simulink model "GPCA_INFUSION_MGR"  (Simulink 8.7)
settings: Solver=VariableStepAuto  StartTime=0.0  StopTime=10.0  RelTol=1e-3
model workspace (MAT data in the model file):
  input_struct.time = [0; 1; 2; 3; 4; 5; 6; 7; 8; 9; 10; 11; 12; 13; 14; 15; 16; 17; 18; 19; 20; 21; 22; 23; 24; 25; 26; 27; 28; 29; 30; 31; 32; 33; 34; 35; 36; 37; 38; 39; 40; 41; 42; 43; 44; 45; 46; 47; 48; 49; 50; 51; 52; 53; 54; 55; 56; 57; 58; 59; 60; 61; 62; 63; 64; 65; 66; 67; 68; 69; 70; 71; 72; 73; 74; 75; 76; 77; 78; 79; 80; 81; 82; 83; 84; 85; 86; 87; 88; 89; 90; 91; 92; 93; 94; 95; 96; 97; 98; 99; 100]
  input_struct.signals(1).name = 'Sys_On'
  input_struct.signals(1).values = [1; 1; 1; 1; 1; 1; 1; 1; 1; 1; 1; 1; 1; 1; 1; 1; 1; 1; 1; 1; 1; 1; 1; 1; 1; 1; 1; 1; 1; 1; 1; 1; 1; 1; 1; 1; 1; 1; 1; 1; 1; 1; 1; 1; 1; 1; 1; 1; 1; 1; 1; 1; 1; 1; 1; 1; 1; 1; 1; 1; 1; 1; 1; 1; 1; 1; 1; 1; 1; 1; 1; 1; 1; 1; 1; 1; 1; 1; 1; 1; 1; 1; 1; 1; 1; 1; 1; 1; 1; 1; 1; 1; 1; 1; 1; 1; 1; 1; 1; 1; 1]
  input_struct.signals(1).dimensions = 1
  input_struct.signals(2).name = 'Infusion_initial'
  input_struct.signals(2).values = [1; 1; 1; 1; 1; 1; 1; 1; 1; 1; 1; 1; 1; 1; 1; 1; 1; 1; 1; 1; 1; 1; 1; 1; 1; 1; 1; 1; 1; 1; 1; 1; 1; 1; 1; 1; 1; 1; 1; 1; 1; 1; 1; 1; 1; 1; 1; 1; 1; 1; 1; 1; 1; 1; 1; 1; 1; 1; 1; 1; 1; 1; 1; 1; 1; 1; 1; 1; 1; 1; 1; 1; 1; 1; 1; 1; 1; 1; 1; 1; 1; 1; 1; 1; 1; 1; 1; 1; 1; 1; 1; 1; 1; 1; 1; 1; 1; 1; 1; 1; 1]
  input_struct.signals(2).dimensions = 1
  input_struct.signals(3).name = 'In3'
  input_struct.signals(3).values = [1; 1; 1; 1; 1; 1; 1; 1; 1; 1; 1; 1; 1; 1; 1; 1; 1; 1; 1; 1; 1; 1; 1; 1; 1; 1; 1; 1; 1; 1; 1; 1; 1; 1; 1; 1; 1; 1; 1; 1; 1; 1; 1; 1; 1; 1; 1; 1; 1; 1; 1; 1; 1; 1; 1; 1; 1; 1; 1; 1; 1; 1; 1; 1; 1; 1; 1; 1; 1; 1; 1; 1; 1; 1; 1; 1; 1; 1; 1; 1; 1; 1; 1; 1; 1; 1; 1; 1; 1; 1; 1; 1; 1; 1; 1; 1; 1; 1; 1; 1; 1]
  input_struct.signals(3).dimensions = 1
  input_struct.signals(4).name = 'In4'
  input_struct.signals(4).values = [1; 1; 1; 1; 1; 1; 1; 1; 1; 1; 1; 1; 1; 1; 1; 1; 1; 1; 1; 1; 1; 1; 1; 1; 1; 1; 1; 1; 1; 1; 1; 1; 1; 1; 1; 1; 1; 1; 1; 1; 1; 1; 1; 1; 1; 1; 1; 1; 1; 1; 1; 1; 1; 1; 1; 1; 1; 1; 1; 1; 1; 1; 1; 1; 1; 1; 1; 1; 1; 1; 1; 1; 1; 1; 1; 1; 1; 1; 1; 1; 1; 1; 1; 1; 1; 1; 1; 1; 1; 1; 1; 1; 1; 1; 1; 1; 1; 1; 1; 1; 1]
  input_struct.signals(4).dimensions = 1
  input_struct.signals(5).name = 'In5'
  input_struct.signals(5).values = [1; 1; 1; 1; 1; 1; 1; 1; 1; 1; 1; 1; 1; 1; 1; 1; 1; 1; 1; 1; 1; 1; 1; 1; 1; 1; 1; 1; 1; 1; 1; 1; 1; 1; 1; 1; 1; 1; 1; 1; 1; 1; 1; 1; 1; 1; 1; 1; 1; 1; 1; 1; 1; 1; 1; 1; 1; 1; 1; 1; 1; 1; 1; 1; 1; 1; 1; 1; 1; 1; 1; 1; 1; 1; 1; 1; 1; 1; 1; 1; 1; 1; 1; 1; 1; 1; 1; 1; 1; 1; 1; 1; 1; 1; 1; 1; 1; 1; 1; 1; 1]
  input_struct.signals(5).dimensions = 1
  input_struct.signals(6).name = 'In6'
  input_struct.signals(6).values = [44; 62; 24; 71; 99; 17; 64; 65; 64; 99; 39; 27; 46; 12; 36; 79; 31; 74; 65; 84; 53; 39; 62; 61; 54; 74; 38; 13; 37; 82; 90; 35; 2; 3; 85; 94; 77; 97; 50; 56; 66; 98; 91; 3; 58; 73; 16; 5; 54; 4; 50; 22; 48; 66; 5; 86; 4; 65; 51; 58; 88; 19; 21; 14; 83; 74; 90; 16; 43; 63; 60; 30; 79; 39; 99; 21; 78; 85; 47; 68; 80; 24; 76; 93; 100; 89; 51; 1; 2; 10; 79; 56; 72; 23; 2; 13; 64; 2; 95; 100; 38]
  input_struct.signals(6).dimensions = 1
  input_struct.signals(7).name = 'In7'
  input_struct.signals(7).values = [90; 60; 84; 49; 6; 47; 32; 92; 90; 66; 25; 24; 55; 40; 76; 40; 27; 35; 94; 38; 49; 24; 54; 22; 30; 54; 51; 50; 92; 74; 90; 81; 45; 24; 7; 29; 44; 46; 98; 93; 60; 59; 12; 40; 95; 22; 18; 35; 63; 44; 42; 29; 91; 69; 11; 9; 2; 92; 37; 43; 58; 19; 3; 66; 46; 20; 20; 70; 75; 55; 53; 41; 56; 74; 30; 79; 8; 48; 40; 92; 43; 95; 41; 25; 88; 50; 43; 56; 25; 26; 21; 59; 84; 86; 65; 99; 98; 69; 79; 35; 79]
  input_struct.signals(7).dimensions = 1
  input_struct.signals(8).name = 'In8'
  input_struct.signals(8).values = [4.63973383023; 35.2832639735; 35.6997824976; 12.9735038436; 98.2246278024; 41.5753843769; 40.648526584; 78.2690731191; 43.3204076201; 57.6278133584; 65.0468332085; 3.301078952; 40.4011686703; 95.8944237105; 59.5519789208; 93.3078447207; 93.7040801805; 75.5739132103; 53.8914185396; 82.4291331591; 1.07468467942; 74.6518961279; 10.3034771476; 4.84107839062; 18.5691118817; 47.2839709594; 0.963562412951; 85.8180487504; 47.3489526284; 14.9934750248; 24.5454645634; 5.6791143473; 20.524479776; 46.5489139189; 46.0975178173; 35.1056074586; 44.1002771924; 32.9407034078; 57.2097266663; 99.2353294257; 71.7850824726; 36.0995549494; 57.2728531087; 38.0334616232; 37.2083265954; 42.4274644079; 74.3126890424; 36.008048598; 62.64892526; 85.2869697994; 12.0024751155; 17.4342661023; 95.0627797395; 97.7501474465; 25.200487502; 28.4620466338; 83.8286322237; 80.2100740647; 36.9961325274; 36.2810980898; 27.1741280369; 25.946930682; 99.4394376478; 4.6263321519; 67.6333122761; 50.1684647694; 11.3288004525; 46.1314661009; 71.8630508731; 96.0602806974; 52.8900107169; 93.5416699007; 98.9586946718; 46.5715874257; 36.3796463512; 9.03358580397; 84.4203757713; 41.3706063981; 75.7358446323; 55.4033391719; 47.6240269519; 26.6590463476; 13.5277473048; 7.77007824224; 84.6593448102; 33.7042967675; 67.3993808562; 10.4432752721; 58.7365871172; 11.4802921597; 24.9345347125; 41.4172719483; 71.5466741055; 86.9670580513; 81.5427904751; 23.2449226705; 34.6335232103; 96.0612364005; 30.1312799866; 15.4196271404; 74.4436488973]
  input_struct.signals(8).dimensions = 1
  input_struct.signals(9).name = 'In9'
  input_struct.signals(9).values = [29; 33; 1; 57; 45; 17; 71; 55; 26; 40; 25; 59; 6; 61; 4; 87; 35; 12; 60; 64; 79; 74; 80; 65; 92; 61; 74; 72; 69; 92; 97; 33; 10; 81; 69; 18; 49; 94; 14; 66; 20; 63; 63; 45; 66; 45; 86; 71; 43; 63; 65; 89; 100; 73; 51; 5; 11; 86; 92; 68; 47; 97; 8; 39; 2; 60; 57; 2; 59; 37; 3; 98; 14; 56; 87; 69; 4; 45; 44; 77; 100; 26; 89; 5; 34; 73; 50; 55; 23; 13; 49; 88; 65; 45; 14; 15; 99; 98; 43; 76; 56]
  input_struct.signals(9).dimensions = 1
  input_struct.signals(10).name = 'In10'
  input_struct.signals(10).values = [75.6654394055; 97.5920093113; 4.18740489107; 35.1003499457; 47.6647962675; 17.4935331391; 35.5904543428; 88.8469466736; 6.915304919; 9.27474343383; 20.580418117; 61.5198979774; 27.3432050518; 74.7785372302; 30.5726330316; 76.5444360829; 25.2885731381; 67.1015975406; 13.1914107685; 94.2448397517; 44.4583183004; 35.7995338956; 16.9800958046; 49.9074065297; 45.2166200379; 6.62159801851; 88.788167464; 90.7784125901; 78.2654328509; 47.1943559213; 79.6142303751; 87.5647388455; 67.2251562171; 7.03827356925; 12.4471905164; 42.5366183349; 78.2665768727; 58.9146545218; 47.2135906387; 3.37884713121; 18.0073535626; 93.1819658789; 59.0764009202; 50.63355074; 21.8438856709; 95.205103594; 36.2259513867; 45.8546754703; 83.0810137982; 79.0665029294; 44.1022733276; 62.4033793782; 95.5508256318; 66.3478658469; 26.6490943364; 72.3154840215; 56.1077886344; 97.2980667354; 30.0872644671; 49.7020498287; 28.3954108418; 7.42080047907; 11.1397187358; 7.53069359706; 99.6192027606; 59.9597679943; 78.8968013382; 86.1268639612; 82.7068266283; 93.6923731938; 3.58534605987; 13.9710786829; 72.5442080874; 87.2094169044; 37.4103271527; 21.6187517238; 57.6010099173; 2.56467550787; 4.35049245994; 93.3449284046; 40.1651928267; 78.4920768198; 24.2628568325; 60.8542724961; 89.3183909504; 62.9419861275; 92.4146871352; 99.5804571701; 15.0089872708; 2.47968997642; 91.1264097869; 14.7997458476; 8.99430572891; 71.5693599151; 17.5014408721; 15.9721590177; 47.8932143834; 94.8731651593; 74.1070141458; 67.2333462131; 7.03452477692]
  input_struct.signals(10).dimensions = 1
  input_struct.signals(11).name = 'In11'
  input_struct.signals(11).values = [30.6105485336; 93.6833055516; 85.6937003671; 89.0847380737; 58.8586918838; 16.2586327547; 17.6045119807; 74.7563614666; 94.5285815976; 65.7979789003; 54.3831976949; 59.7653088285; 23.4602892008; 81.9767731385; 78.8495533289; 58.9059613176; 43.6259778173; 54.973942777; 35.2968705936; 99.5791193529; 36.4963600016; 96.6174491518; 2.47408729527; 77.7839114133; 44.0182119351; 63.0499928301; 31.4024696203; 92.1815284508; 22.3324620519; 37.4486271858; 30.8144382373; 3.78224741229; 60.5169674512; 83.586436936; 58.8252232814; 36.3454795409; 13.988518362; 11.6533721537; 98.1217434069; 54.169234903; 8.65099084385; 25.6096227789; 20.9775010836; 31.4609803605; 90.3751596102; 52.0696307127; 16.2236010012; 14.3612207513; 6.40530754781; 85.4645458624; 97.4456785593; 92.9025103555; 40.9520221274; 90.1611220035; 48.4497228782; 46.9673840237; 16.7828198886; 8.28584731024; 63.3161255034; 31.0978917444; 46.6354034749; 21.1069421813; 0.14457196441; 79.7611265023; 36.8047426089; 1.513757221; 71.497846647; 21.8578762078; 68.8717269625; 24.6007221266; 26.6084854589; 13.2070823774; 34.4210335433; 75.4389983788; 88.9238646635; 71.0436376648; 24.647502524; 45.1389348495; 93.1224274285; 61.5667580202; 25.8289980493; 63.1103174057; 69.5532194169; 40.3659878092; 19.3481857413; 30.7074224713; 69.2954513388; 63.0359565476; 24.9823988841; 4.34220177336; 53.1451453615; 17.6201447979; 52.1902037473; 87.1282135693; 61.3612826085; 27.1432121467; 85.453961022; 15.7460139606; 25.941863813; 67.0580480613; 22.5957392867]
  input_struct.signals(11).dimensions = 1
  input_struct.signals(12).name = 'In12'
  input_struct.signals(12).values = [83; 33; 49; 77; 74; 64; 25; 74; 34; 31; 13; 2; 93; 92; 39; 71; 68; 13; 21; 91; 90; 38; 26; 61; 63; 2; 82; 52; 91; 12; 95; 93; 10; 42; 33; 85; 95; 73; 69; 65; 32; 74; 16; 77; 10; 97; 61; 90; 20; 99; 25; 23; 41; 79; 84; 41; 41; 78; 25; 87; 69; 98; 19; 22; 32; 76; 37; 61; 39; 56; 39; 67; 2; 82; 35; 72; 96; 51; 67; 43; 85; 66; 51; 37; 69; 10; 5; 87; 66; 62; 43; 51; 17; 10; 69; 15; 53; 1; 43; 23; 66]
  input_struct.signals(12).dimensions = 1
  input_struct.signals(13).name = 'In13'
  input_struct.signals(13).values = [50.310189638; 60.0057239808; 20.017365886; 13.7401018724; 2.37890286344; 93.9542698221; 69.550132379; 55.4233183009; 29.5414289119; 4.26317475057; 85.3760208334; 59.6682100841; 1.85267796429; 93.3190961871; 0.978832426687; 64.0955539628; 78.8685383549; 52.6502944231; 29.1248417281; 62.8328540884; 42.5468671552; 54.6370363273; 19.0797083319; 74.448883701; 21.2856219278; 10.0122455877; 89.6384986298; 82.2336975388; 88.278375005; 8.81242954122; 70.0187647741; 17.022422373; 83.3044271053; 72.8057084722; 77.5893015136; 76.3495251449; 5.70994655747; 60.9847721619; 89.8471800448; 51.6130724509; 50.6171538067; 25.5616556411; 97.1603134959; 58.1123922451; 96.8386414337; 4.14383729209; 18.8628229362; 51.9760059068; 64.0853919663; 34.0731322525; 64.8329819208; 35.5437965546; 85.0430024041; 54.2804681241; 67.3080087461; 25.6572579313; 12.1338276708; 4.06064458603; 88.7943133089; 75.3187315832; 80.2079185026; 44.1405626647; 7.51725857162; 15.4229697288; 24.7244148394; 7.92259868541; 85.3159563134; 15.7176855291; 61.6662683689; 52.8449944459; 19.1219823356; 75.9750760227; 61.4998425493; 15.2063606777; 45.4637446858; 68.2097599809; 28.1259121576; 62.4863120815; 94.1730122601; 56.6803336047; 69.3115599105; 97.8586411034; 89.9117378675; 64.8479896015; 98.2920814945; 16.381496818; 50.9786857228; 62.7348429656; 80.0000906333; 41.7769086107; 5.48344318938; 51.9144193651; 13.4532135688; 36.6974434645; 69.6620887403; 12.9583524717; 78.5849529987; 5.03089735964; 81.5615519701; 86.6938862459; 19.6896453654]
  input_struct.signals(13).dimensions = 1
  input_struct.signals(14).name = 'In14'
  input_struct.signals(14).values = [60.7393801127; 99.6679751886; 4.23743274601; 13.8823003129; 22.2953974091; 58.3010477964; 67.1106486856; 72.3195985118; 50.4438512986; 64.4630262831; 3.6369340676; 19.3851825335; 74.9545712103; 30.8178375845; 74.9052151825; 85.2037321352; 9.93554763828; 59.7778198788; 72.0602255764; 56.8713832115; 23.5110091085; 91.0636226409; 95.0619757095; 51.631529482; 70.7088130257; 79.879519294; 19.9689366653; 10.684051545; 61.8574843316; 2.22239407823; 3.75620436883; 11.5364121588; 81.8697240446; 37.6899225803; 22.9156312136; 36.8139913037; 17.4540423871; 77.4779638833; 33.0030614354; 31.5780139928; 72.4586900626; 58.4954983442; 77.7755524267; 35.9576387651; 18.4733001916; 57.3689108129; 48.3094584565; 42.1626940454; 31.7325192381; 97.2571507193; 25.8222640837; 56.7099899646; 35.2066904741; 31.202960892; 0.939760275739; 66.8127492036; 88.5687680497; 42.1317726472; 85.8580052735; 94.7992491693; 37.6106774797; 20.329324849; 17.9169495241; 30.6294083341; 85.0311935666; 52.5602531045; 82.844225188; 10.6876458874; 61.71420317; 56.6826518566; 26.0936156907; 0.230811043294; 28.725506288; 82.1270082457; 89.511540468; 99.5807909606; 0.843840180703; 73.284323844; 8.46172679425; 63.3348568099; 80.5086425609; 82.9964886435; 56.7221449724; 26.0043390493; 78.4532049402; 16.9205334021; 27.4258345175; 0.490319428856; 39.7561240528; 2.65515532308; 85.469904981; 20.4891689163; 86.0350581098; 5.61247088055; 22.3511772366; 4.52805178084; 75.0991773113; 69.805637993; 91.8787889121; 90.8922604332; 80.5523856545]
  input_struct.signals(14).dimensions = 1
  input_struct.signals(15).name = 'In15'
  input_struct.signals(15).values = [100; 81; 33; 3; 74; 48; 40; 87; 6; 39; 15; 5; 70; 92; 39; 25; 91; 71; 90; 95; 94; 100; 40; 66; 83; 63; 71; 49; 51; 78; 5; 91; 74; 62; 76; 29; 21; 66; 93; 81; 36; 28; 75; 73; 86; 92; 27; 69; 62; 8; 19; 34; 32; 43; 9; 56; 67; 12; 32; 99; 89; 3; 87; 25; 44; 14; 22; 78; 9; 41; 60; 20; 70; 60; 47; 25; 42; 78; 4; 61; 8; 42; 99; 85; 6; 73; 12; 49; 87; 2; 82; 79; 20; 92; 69; 89; 72; 49; 84; 10; 3]
  input_struct.signals(15).dimensions = 1
  input_struct.signals(16).name = 'In16'
  input_struct.signals(16).values = [34; 49; 23; 56; 69; 84; 90; 44; 40; 45; 31; 45; 97; 47; 50; 3; 20; 90; 39; 11; 35; 18; 25; 65; 98; 93; 6; 91; 19; 100; 33; 23; 95; 82; 93; 72; 88; 87; 36; 14; 81; 69; 44; 95; 96; 4; 28; 7; 83; 40; 59; 35; 98; 61; 67; 87; 43; 8; 88; 70; 85; 68; 71; 90; 59; 33; 100; 21; 29; 84; 78; 21; 77; 62; 97; 51; 48; 59; 98; 35; 27; 59; 75; 9; 38; 9; 32; 46; 17; 6; 45; 29; 20; 51; 2; 84; 21; 43; 74; 53; 27]
  input_struct.signals(16).dimensions = 1
  input_struct.signals(17).name = 'In17'
  input_struct.signals(17).values = [77; 96; 12; 3; 43; 7; 13; 10; 24; 22; 61; 40; 73; 97; 76; 8; 87; 37; 80; 79; 34; 95; 83; 63; 30; 62; 99; 35; 24; 1; 91; 63; 79; 75; 62; 19; 85; 72; 66; 62; 88; 80; 73; 41; 100; 63; 36; 19; 33; 26; 95; 90; 99; 96; 88; 17; 15; 65; 80; 8; 25; 2; 24; 26; 92; 37; 4; 66; 82; 9; 2; 37; 42; 42; 47; 47; 55; 54; 51; 79; 29; 56; 58; 21; 56; 22; 55; 7; 87; 21; 24; 39; 29; 76; 32; 11; 81; 26; 51; 4; 63]
  input_struct.signals(17).dimensions = 1
  input_struct.signals(18).name = 'In18'
  input_struct.signals(18).values = [39; 31; 34; 94; 47; 1; 73; 40; 3; 64; 44; 60; 62; 46; 5; 72; 75; 41; 6; 95; 88; 83; 45; 89; 86; 65; 51; 8; 37; 24; 87; 64; 74; 16; 95; 41; 62; 80; 69; 1; 51; 99; 1; 5; 11; 61; 5; 43; 36; 70; 37; 33; 68; 59; 25; 38; 21; 26; 85; 43; 66; 54; 94; 34; 37; 75; 87; 3; 85; 81; 55; 44; 61; 34; 78; 10; 46; 77; 63; 1; 2; 46; 23; 38; 45; 7; 37; 38; 31; 92; 48; 19; 30; 83; 62; 67; 62; 27; 88; 1; 37]
  input_struct.signals(18).dimensions = 1
  input_struct.signals(19).name = 'In19'
  input_struct.signals(19).values = [1; 1; 1; 1; 1; 1; 1; 1; 1; 1; 1; 1; 1; 1; 1; 1; 1; 1; 1; 1; 1; 1; 1; 1; 1; 1; 1; 1; 1; 1; 1; 1; 1; 1; 1; 1; 1; 1; 1; 1; 1; 1; 1; 1; 1; 1; 1; 1; 1; 1; 1; 1; 1; 1; 1; 1; 1; 1; 1; 1; 1; 1; 1; 1; 1; 1; 1; 1; 1; 1; 1; 1; 1; 1; 1; 1; 1; 1; 1; 1; 1; 1; 1; 1; 1; 1; 1; 1; 1; 1; 1; 1; 1; 1; 1; 1; 1; 1; 1; 1; 1]
  input_struct.signals(19).dimensions = 1
  input_struct.signals(20).name = 'In20'
  input_struct.signals(20).values = [45; 15; 66; 68; 75; 31; 81; 30; 28; 28; 77; 32; 36; 68; 4; 16; 43; 22; 77; 65; 84; 21; 44; 74; 11; 45; 50; 70; 94; 16; 6; 61; 25; 56; 68; 47; 66; 81; 86; 72; 27; 30; 19; 60; 78; 10; 41; 64; 77; 52; 5; 45; 79; 100; 85; 6; 77; 73; 76; 21; 33; 60; 98; 46; 50; 98; 77; 98; 21; 4; 16; 72; 78; 65; 34; 66; 5; 87; 11; 95; 38; 14; 32; 90; 79; 20; 18; 90; 78; 80; 22; 20; 65; 12; 51; 69; 16; 38; 81; 91; 17]
  input_struct.signals(20).dimensions : numeric (value not decoded)
libraries: simulink x12
settings Model: Creator=bourbouh  LastModifiedBy=bourbouh
settings DataIOCC: LimitDataPoints=off  SaveFormat=Dataset
settings DebuggingCC: UnderspecifiedInitializationDetection=Simplified  MergeDetectMultiDrivingBlocksExec=error
settings HardwareCC: ProdBitPerPointer=64  ProdLargestAtomicFloat=Float  ProdIntDivRoundTo=Zero  ProdEndianess=LittleEndian  ProdWordSize=64  ProdHWDeviceType=Intel->x86-64 (Windows64)
settings ModelReferenceCC: PropagateSignalLabelsOutOfModel=on
settings ConfigComp: CovModelRefEnable=off

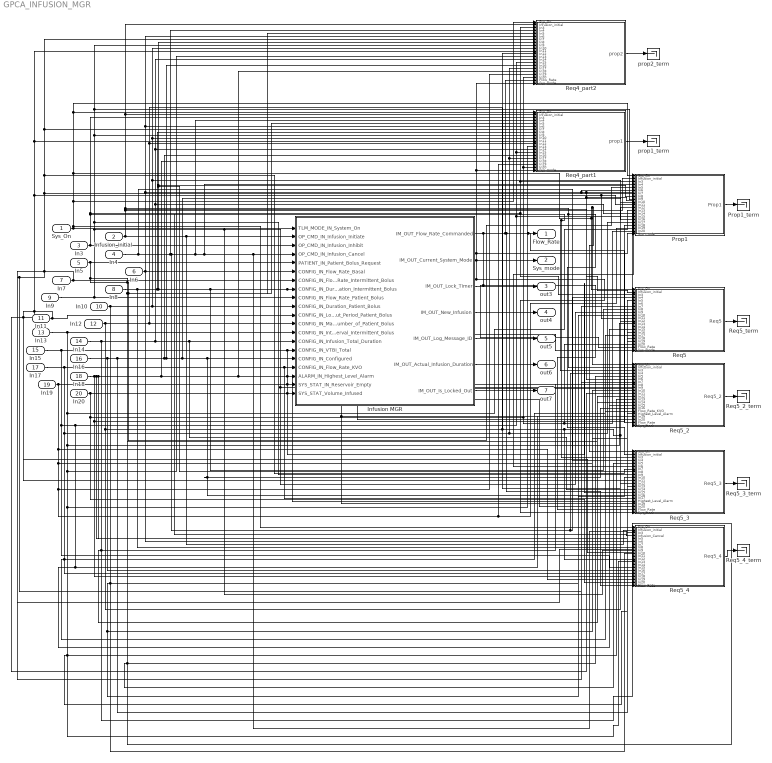
== system GPCA_INFUSION_MGR ==
  Sys_On : Inport
  Infusion_initial : Inport  Port=2
  In3 : Inport  Port=3
  In4 : Inport  Port=4
  In5 : Inport  Port=5
  In6 : Inport  Port=6
  In7 : Inport  Port=7
  In8 : Inport  Port=8
  In9 : Inport  Port=9
  In10 : Inport  Port=10
  In11 : Inport  Port=11
  In12 : Inport  Port=12
  In13 : Inport  Port=13
  In14 : Inport  Port=14
  In15 : Inport  Port=15
  In16 : Inport  Port=16
  In17 : Inport  Port=17
  In18 : Inport  Port=18
  In19 : Inport  Port=19
  In20 : Inport  Port=20
  Infusion MGR : Stateflow chart  TreatAsAtomicUnit=on
  Prop1 : Subsystem  TreatAsAtomicUnit=on  mask(Observer){AnnotationType=ensures, ObserverType=[]}
      mask prompts: AnnotationType "Type of annotation (pre/post...)"; ObserverType "Observer type"
      mask help:
      | Set an observer for the system.
      | The annotation type parameter sets the type of observer:
      | - requires : pre-condition
      | - ensures : post-condition
      | - assert : an assertion
      | - observer : the observer computes a special type of properties
      mask TypeOptions AnnotationType: ensures | requires | assert | observer
      mask Callback AnnotationType:
      | paramStr = get_param(gcb, 'MaskValues');
      | if strcmp(paramStr{1}(1),'o')
      | set_param(gcb,'MaskVisibilities',{'on';'on'});
      | paramStr{2} = 'ellipsoid';
      | set_param(gcb,'MaskValues',paramStr);
      | else
      | set_param(gcb,'MaskVisibilities',{'on';'off'});
      | end
      | clear paramStr;
      mask Callback ObserverType:
      | paramStr = get_param(gcb, 'MaskValues');
      | if strcmp(paramStr{1}(1),'o')
      | set_param(gcb,'MaskVisibilities',{'on';'on'});
      | paramStr{2} = 'ellipsoid';
      | set_param(gcb,'MaskValues',paramStr);
      | else
      | set_param(gcb,'MaskVisibilities',{'on';'off'});
      | end
      | clear paramStr;
      mask Display:
      | color('black')
      | text(0.5, 0.5, ['Property: ''' get_param(gcb,'name') ''''], 'horizontalAlignment', 'center');
      | text(0.99, 0.03, '{\bf\fontsize{12}SAFE}', 'hor', 'right', 'ver', 'bottom', 'texmode', 'on');
  Prop1_term : Terminator
  Req4_part1 : Subsystem  TreatAsAtomicUnit=on  mask(Observer){AnnotationType=ensures, ObserverType=[]}
      mask prompts: AnnotationType "Type of annotation (pre/post...)"; ObserverType "Observer type"
      mask help:
      | Set an observer for the system.
      | The annotation type parameter sets the type of observer:
      | - requires : pre-condition
      | - ensures : post-condition
      | - assert : an assertion
      | - observer : the observer computes a special type of properties
      mask TypeOptions AnnotationType: ensures | requires | assert | observer
      mask Callback AnnotationType:
      | paramStr = get_param(gcb, 'MaskValues');
      | if strcmp(paramStr{1}(1),'o')
      | set_param(gcb,'MaskVisibilities',{'on';'on'});
      | paramStr{2} = 'ellipsoid';
      | set_param(gcb,'MaskValues',paramStr);
      | else
      | set_param(gcb,'MaskVisibilities',{'on';'off'});
      | end
      | clear paramStr;
      mask Callback ObserverType:
      | paramStr = get_param(gcb, 'MaskValues');
      | if strcmp(paramStr{1}(1),'o')
      | set_param(gcb,'MaskVisibilities',{'on';'on'});
      | paramStr{2} = 'ellipsoid';
      | set_param(gcb,'MaskValues',paramStr);
      | else
      | set_param(gcb,'MaskVisibilities',{'on';'off'});
      | end
      | clear paramStr;
      mask Display:
      | color('black')
      | text(0.5, 0.5, ['Property: ''' get_param(gcb,'name') ''''], 'horizontalAlignment', 'center');
      | text(0.99, 0.03, '{\bf\fontsize{12}SAFE}', 'hor', 'right', 'ver', 'bottom', 'texmode', 'on');
  Req4_part2 : Subsystem  TreatAsAtomicUnit=on  mask(Observer){AnnotationType=ensures, ObserverType=[]}
      mask prompts: AnnotationType "Type of annotation (pre/post...)"; ObserverType "Observer type"
      mask help:
      | Set an observer for the system.
      | The annotation type parameter sets the type of observer:
      | - requires : pre-condition
      | - ensures : post-condition
      | - assert : an assertion
      | - observer : the observer computes a special type of properties
      mask TypeOptions AnnotationType: ensures | requires | assert | observer
      mask Callback AnnotationType:
      | paramStr = get_param(gcb, 'MaskValues');
      | if strcmp(paramStr{1}(1),'o')
      | set_param(gcb,'MaskVisibilities',{'on';'on'});
      | paramStr{2} = 'ellipsoid';
      | set_param(gcb,'MaskValues',paramStr);
      | else
      | set_param(gcb,'MaskVisibilities',{'on';'off'});
      | end
      | clear paramStr;
      mask Callback ObserverType:
      | paramStr = get_param(gcb, 'MaskValues');
      | if strcmp(paramStr{1}(1),'o')
      | set_param(gcb,'MaskVisibilities',{'on';'on'});
      | paramStr{2} = 'ellipsoid';
      | set_param(gcb,'MaskValues',paramStr);
      | else
      | set_param(gcb,'MaskVisibilities',{'on';'off'});
      | end
      | clear paramStr;
      mask Display:
      | color('black')
      | text(0.5, 0.5, ['Property: ''' get_param(gcb,'name') ''''], 'horizontalAlignment', 'center');
      | text(0.99, 0.03, '{\bf\fontsize{12}TIMEOUT}', 'hor', 'right', 'ver', 'bottom', 'texmode', 'on');
  Req5 : Subsystem  TreatAsAtomicUnit=on  mask(Observer){AnnotationType=ensures, ObserverType=[]}
      mask prompts: AnnotationType "Type of annotation (pre/post...)"; ObserverType "Observer type"
      mask help:
      | Set an observer for the system.
      | The annotation type parameter sets the type of observer:
      | - requires : pre-condition
      | - ensures : post-condition
      | - assert : an assertion
      | - observer : the observer computes a special type of properties
      mask TypeOptions AnnotationType: ensures | requires | assert | observer
      mask Callback AnnotationType:
      | paramStr = get_param(gcb, 'MaskValues');
      | if strcmp(paramStr{1}(1),'o')
      | set_param(gcb,'MaskVisibilities',{'on';'on'});
      | paramStr{2} = 'ellipsoid';
      | set_param(gcb,'MaskValues',paramStr);
      | else
      | set_param(gcb,'MaskVisibilities',{'on';'off'});
      | end
      | clear paramStr;
      mask Callback ObserverType:
      | paramStr = get_param(gcb, 'MaskValues');
      | if strcmp(paramStr{1}(1),'o')
      | set_param(gcb,'MaskVisibilities',{'on';'on'});
      | paramStr{2} = 'ellipsoid';
      | set_param(gcb,'MaskValues',paramStr);
      | else
      | set_param(gcb,'MaskVisibilities',{'on';'off'});
      | end
      | clear paramStr;
      mask Display:
      | color('black')
      | text(0.5, 0.5, ['Property: ''' get_param(gcb,'name') ''''], 'horizontalAlignment', 'center');
      | text(0.99, 0.03, '{\bf\fontsize{12}SAFE}', 'hor', 'right', 'ver', 'bottom', 'texmode', 'on');
  Req5_2 : Subsystem  TreatAsAtomicUnit=on  mask(Observer){AnnotationType=ensures, ObserverType=[]}
      mask prompts: AnnotationType "Type of annotation (pre/post...)"; ObserverType "Observer type"
      mask help:
      | Set an observer for the system.
      | The annotation type parameter sets the type of observer:
      | - requires : pre-condition
      | - ensures : post-condition
      | - assert : an assertion
      | - observer : the observer computes a special type of properties
      mask TypeOptions AnnotationType: ensures | requires | assert | observer
      mask Callback AnnotationType:
      | paramStr = get_param(gcb, 'MaskValues');
      | if strcmp(paramStr{1}(1),'o')
      | set_param(gcb,'MaskVisibilities',{'on';'on'});
      | paramStr{2} = 'ellipsoid';
      | set_param(gcb,'MaskValues',paramStr);
      | else
      | set_param(gcb,'MaskVisibilities',{'on';'off'});
      | end
      | clear paramStr;
      mask Callback ObserverType:
      | paramStr = get_param(gcb, 'MaskValues');
      | if strcmp(paramStr{1}(1),'o')
      | set_param(gcb,'MaskVisibilities',{'on';'on'});
      | paramStr{2} = 'ellipsoid';
      | set_param(gcb,'MaskValues',paramStr);
      | else
      | set_param(gcb,'MaskVisibilities',{'on';'off'});
      | end
      | clear paramStr;
      mask Display:
      | color('black')
      | text(0.5, 0.5, ['Property: ''' get_param(gcb,'name') ''''], 'horizontalAlignment', 'center');
      | text(0.99, 0.03, '{\bf\fontsize{12}SAFE}', 'hor', 'right', 'ver', 'bottom', 'texmode', 'on');
  Req5_2_term : Terminator
  Req5_3 : Subsystem  TreatAsAtomicUnit=on  mask(Observer){AnnotationType=ensures, ObserverType=[]}
      mask prompts: AnnotationType "Type of annotation (pre/post...)"; ObserverType "Observer type"
      mask help:
      | Set an observer for the system.
      | The annotation type parameter sets the type of observer:
      | - requires : pre-condition
      | - ensures : post-condition
      | - assert : an assertion
      | - observer : the observer computes a special type of properties
      mask TypeOptions AnnotationType: ensures | requires | assert | observer
      mask Callback AnnotationType:
      | paramStr = get_param(gcb, 'MaskValues');
      | if strcmp(paramStr{1}(1),'o')
      | set_param(gcb,'MaskVisibilities',{'on';'on'});
      | paramStr{2} = 'ellipsoid';
      | set_param(gcb,'MaskValues',paramStr);
      | else
      | set_param(gcb,'MaskVisibilities',{'on';'off'});
      | end
      | clear paramStr;
      mask Callback ObserverType:
      | paramStr = get_param(gcb, 'MaskValues');
      | if strcmp(paramStr{1}(1),'o')
      | set_param(gcb,'MaskVisibilities',{'on';'on'});
      | paramStr{2} = 'ellipsoid';
      | set_param(gcb,'MaskValues',paramStr);
      | else
      | set_param(gcb,'MaskVisibilities',{'on';'off'});
      | end
      | clear paramStr;
      mask Display:
      | color('black')
      | text(0.5, 0.5, ['Property: ''' get_param(gcb,'name') ''''], 'horizontalAlignment', 'center');
      | text(0.99, 0.03, '{\bf\fontsize{12}TIMEOUT}', 'hor', 'right', 'ver', 'bottom', 'texmode', 'on');
  Req5_3_term : Terminator
  Req5_4 : Subsystem  TreatAsAtomicUnit=on  mask(Observer){AnnotationType=ensures, ObserverType=[]}
      mask prompts: AnnotationType "Type of annotation (pre/post...)"; ObserverType "Observer type"
      mask help:
      | Set an observer for the system.
      | The annotation type parameter sets the type of observer:
      | - requires : pre-condition
      | - ensures : post-condition
      | - assert : an assertion
      | - observer : the observer computes a special type of properties
      mask TypeOptions AnnotationType: ensures | requires | assert | observer
      mask Callback AnnotationType:
      | paramStr = get_param(gcb, 'MaskValues');
      | if strcmp(paramStr{1}(1),'o')
      | set_param(gcb,'MaskVisibilities',{'on';'on'});
      | paramStr{2} = 'ellipsoid';
      | set_param(gcb,'MaskValues',paramStr);
      | else
      | set_param(gcb,'MaskVisibilities',{'on';'off'});
      | end
      | clear paramStr;
      mask Callback ObserverType:
      | paramStr = get_param(gcb, 'MaskValues');
      | if strcmp(paramStr{1}(1),'o')
      | set_param(gcb,'MaskVisibilities',{'on';'on'});
      | paramStr{2} = 'ellipsoid';
      | set_param(gcb,'MaskValues',paramStr);
      | else
      | set_param(gcb,'MaskVisibilities',{'on';'off'});
      | end
      | clear paramStr;
      mask Display:
      | color('black')
      | text(0.5, 0.5, ['Property: ''' get_param(gcb,'name') ''''], 'horizontalAlignment', 'center');
      | text(0.99, 0.03, '{\bf\fontsize{12}SAFE}', 'hor', 'right', 'ver', 'bottom', 'texmode', 'on');
  Req5_4_term : Terminator
  Req5_term : Terminator
  prop1_term : Terminator
  prop2_term : Terminator
  Flow_Rate : Outport
  Sys_mode : Outport  Port=2
  out3 : Outport  Port=3
  out4 : Outport  Port=4
  out5 : Outport  Port=5
  out6 : Outport  Port=6
  out7 : Outport  Port=7
  wires:
  Sys_On/1 -> Req5_3/1(Sys_On), Req5_2/1(Sys_On), Req5/1(Sys_On), Prop1/1(Sys_On), Req4_part1/1(Sys_On), Req4_part2/1(Sys_On), Req5_4/1(Sys_On), Infusion MGR/1(TLM_MODE_IN_System_On)
  Infusion_initial/1 -> Infusion MGR/2(OP_CMD_IN_Infusion_Initiate), Req5_4/2(Infusion_initial), Req4_part2/2(Infusion_initial), Req4_part1/2(Infusion_initial), Req5_3/2(Infusion_initial), Req5_2/2(Infusion_initial), Req5/2(Infusion_initial), Prop1/2(Infusion_initial)
  In3/1 -> Req5_4/3(In3), Prop1/3(In3), Req4_part2/3(In3), Req5/3(In3), Req4_part1/3(In3), Req5_2/3(In3), Req5_3/3(In3), Infusion MGR/3(OP_CMD_IN_Infusion_Inhibit)
  In4/1 -> Req5_4/4(Infusion_Cancel), Infusion MGR/4(OP_CMD_IN_Infusion_Cancel), Prop1/4(In4), Req4_part1/4(In4), Req5_2/4(In4), Req5/4(In4), Req4_part2/4(In4), Req5_3/4(In4)
  In5/1 -> Req5_4/5(In5), Req5_3/5(In5), Req5_2/5(In5), Prop1/5(In5), Req4_part1/5(In5), Req5/5(In5), Req4_part2/5(In5), Infusion MGR/5(PATIENT_IN_Patient_Bolus_Request)
  In6/1 -> Req5/6(In6), Req5_3/6(In6), Req5_2/6(In6), Prop1/6(In6), Req4_part2/6(In6), Req4_part1/6(In6), Infusion MGR/6(CONFIG_IN_Flow_Rate_Basal), Req5_4/6(In6)
  In7/1 -> Req5_4/7(In7), Req5_3/7(In7), Req4_part2/7(In7), Req4_part1/7(In7), Prop1/7(In7), Req5_2/7(In7), Req5/7(In7), Infusion MGR/7(CONFIG_IN_Flow_Rate_Intermittent_Bolus)
  In8/1 -> Prop1/8(In8), Req4_part2/8(In8), Req5_3/8(In8), Req5_2/8(In8), Infusion MGR/8(CONFIG_IN_Duration_Intermittent_Bolus), Req5/8(In8), Req4_part1/8(In8), Req5_4/8(In8)
  In9/1 -> Req5_4/9(In9), Req5_2/9(In9), Req5/9(In9), Prop1/9(In9), Req4_part2/9(In9), Req4_part1/9(In9), Req5_3/9(In9), Infusion MGR/9(CONFIG_IN_Flow_Rate_Patient_Bolus)
  In10/1 -> Req5_4/10(In10), Req5_3/10(In10), Req5_2/10(In10), Req5/10(In10), Req4_part2/10(In10), Req4_part1/10(In10), Prop1/10(In10), Infusion MGR/10(CONFIG_IN_Duration_Patient_Bolus)
  In11/1 -> Req5_4/11(In11), Req5_3/11(In11), Req5_2/11(In11), Prop1/11(In11), Req5/11(In11), Req4_part2/11(In11), Req4_part1/11(In11), Infusion MGR/11(CONFIG_IN_Lockout_Period_Patient_Bolus)
  In12/1 -> Req5_4/12(In12), Req5/12(In12), Prop1/12(In12), Req4_part2/12(In12), Req5_2/12(In12), Req5_3/12(In12), Req4_part1/12(In12), Infusion MGR/12(CONFIG_IN_Max_Number_of_Patient_Bolus)
  In13/1 -> Req5_4/13(In13), Req5_3/13(In13), Req5_2/13(In13), Req4_part1/13(In13), Req4_part2/13(In13), Req5/13(In13), Prop1/13(In13), Infusion MGR/13(CONFIG_IN_Interval_Intermittent_Bolus)
  In14/1 -> Req5_4/14(In14), Req5_2/14(In14), Req5/14(In14), Req5_3/14(In14), Infusion MGR/14(CONFIG_IN_Infusion_Total_Duration), Req4_part2/14(In14), Req4_part1/14(In14), Prop1/14(In14)
  In15/1 -> Req5_4/15(In15), Req5_2/15(In15), Req5/15(In15), Req4_part2/15(In15), Req4_part1/15(In15), Prop1/15(In15), Req5_3/15(In15), Infusion MGR/15(CONFIG_IN_VTBI_Total)
  In16/1 -> Req5_2/16(In16), Req5_3/16(In16), Infusion MGR/16(CONFIG_IN_Configured), Prop1/16(In16), Req4_part2/16(In16), Req4_part1/16(In16), Req5/16(In16), Req5_4/16(In16)
  In17/1 -> Req5_4/17(In17), Req5_2/17(Flow_Rate_KVO), Req5/17(In17), Req4_part2/17(In17), Req4_part1/17(In17), Prop1/17(In17), Infusion MGR/17(CONFIG_IN_Flow_Rate_KVO), Req5_3/17(In17)
  In18/1 -> Req5_4/18(In18), Prop1/18(In18), Req5_3/18(Highest_Level_Alarm), Infusion MGR/18(ALARM_IN_Highest_Level_Alarm), Req4_part2/18(In18), Req4_part1/18(In18), Req5/18(In18), Req5_2/18(Highest_Level_Alarm)
  In19/1 -> Prop1/19(In19), Req4_part1/19(In19), Req4_part2/19(In19), Req5/19(In19), Req5_4/19(In19), Req5_3/19(In19), Req5_2/19(In19), Infusion MGR/19(SYS_STAT_IN_Reservoir_Empty)
  In20/1 -> Req5/20(In20), Prop1/20(In20), Req4_part2/20(In20), Req4_part1/20(In20), Req5_4/20(In20), Req5_3/20(In20), Req5_2/20(In20), Infusion MGR/20(SYS_STAT_Volume_Infused)
  Infusion MGR/2(IM_OUT_Current_System_Mode) -> Req5/22(Sys_mode), Req5_2/22(Sys_mode), Req5_3/22(Sys_mode), Req4_part2/22(Sys_mode), Req4_part1/21(Sys_mode), Prop1/21(Sys_mode), Sys_mode/1
  Infusion MGR/3(IM_OUT_Lock_Timer) -> out3/1
  Infusion MGR/1(IM_OUT_Flow_Rate_Commanded) -> Req5_4/21(Flow_Rate), Req5_2/21(Flow_Rate), Flow_Rate/1, Req4_part2/21(Flow_Rate), Req5/21(Flow_Rate), Req5_3/21(Flow_Rate)
  Infusion MGR/4(IM_OUT_New_Infusion) -> out4/1
  Infusion MGR/5(IM_OUT_Log_Message_ID) -> out5/1
  Infusion MGR/6(IM_OUT_Actual_Infusion_Duration) -> out6/1
  Infusion MGR/7(IM_OUT_Is_Locked_Out) -> out7/1
  Req4_part1/1(prop1) -> prop1_term/1
  Req4_part2/1(prop2) -> prop2_term/1
  Prop1/1(Prop1) -> Prop1_term/1
  Req5/1(Req5) -> Req5_term/1
  Req5_2/1(Req5_2) -> Req5_2_term/1
  Req5_3/1(Req5_3) -> Req5_3_term/1
  Req5_4/1(Req5_4) -> Req5_4_term/1

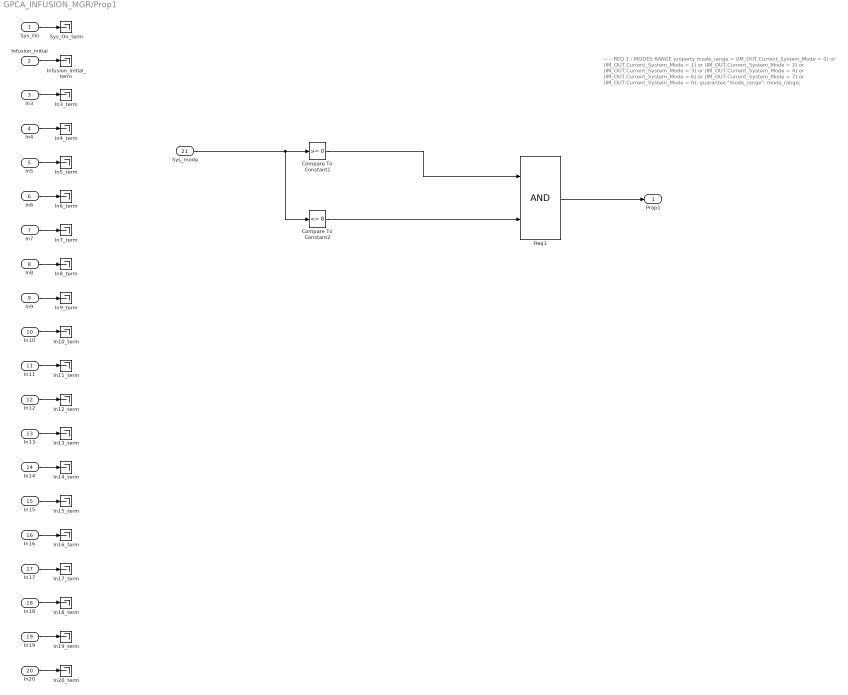
== system GPCA_INFUSION_MGR/Prop1 ==
  note: -- -- REQ 1 : MODES RANGE
      | property mode_range =
      | (IM_OUT.Current_System_Mode = 0) or
      | (IM_OUT.Current_System_Mode = 1) or
      | (IM_OUT.Current_System_Mode = 2) or
      | (IM_OUT.Current_System_Mode = 3) or
      | (IM_OUT.Current_System_Mode = 4) or
      | (IM_OUT.Current_System_Mode = 6) or
      | (IM_OUT.Current_System_Mode = 7) or
      | (IM_OUT.Current_System_Mode = 8);
      | guarantee "mode_range": mode_range;
  Sys_On : Inport
  Infusion_initial : Inport  Port=2
  In3 : Inport  Port=3
  In4 : Inport  Port=4
  In5 : Inport  Port=5
  In6 : Inport  Port=6
  In7 : Inport  Port=7
  In8 : Inport  Port=8
  In9 : Inport  Port=9
  In10 : Inport  Port=10
  In11 : Inport  Port=11
  In12 : Inport  Port=12
  In13 : Inport  Port=13
  In14 : Inport  Port=14
  In15 : Inport  Port=15
  In16 : Inport  Port=16
  In17 : Inport  Port=17
  In18 : Inport  Port=18
  In19 : Inport  Port=19
  In20 : Inport  Port=20
  Sys_mode : Inport  Port=21
  Compare To Constant1 : simulink/Logic and Bit Operations/Compare To Constant  relop=>=  const=0  OutDataTypeStr=boolean
  Compare To Constant2 : simulink/Logic and Bit Operations/Compare To Constant  relop=<=  const=8  OutDataTypeStr=boolean
  In10_term : Terminator
  In11_term : Terminator
  In12_term : Terminator
  In13_term : Terminator
  In14_term : Terminator
  In15_term : Terminator
  In16_term : Terminator
  In17_term : Terminator
  In18_term : Terminator
  In19_term : Terminator
  In20_term : Terminator
  In3_term : Terminator
  In4_term : Terminator
  In5_term : Terminator
  In6_term : Terminator
  In7_term : Terminator
  In8_term : Terminator
  In9_term : Terminator
  Infusion_initial_term : Terminator
  Req1 : Logic  AllPortsSameDT=off  OutDataTypeStr=boolean
  Sys_On_term : Terminator
  Prop1 : Outport
  wires:
  Sys_On/1 -> Sys_On_term/1
  Infusion_initial/1 -> Infusion_initial_term/1
  In3/1 -> In3_term/1
  In4/1 -> In4_term/1
  In5/1 -> In5_term/1
  In6/1 -> In6_term/1
  In7/1 -> In7_term/1
  In8/1 -> In8_term/1
  In9/1 -> In9_term/1
  In10/1 -> In10_term/1
  In11/1 -> In11_term/1
  In12/1 -> In12_term/1
  In13/1 -> In13_term/1
  In14/1 -> In14_term/1
  In15/1 -> In15_term/1
  In16/1 -> In16_term/1
  In17/1 -> In17_term/1
  In18/1 -> In18_term/1
  In19/1 -> In19_term/1
  In20/1 -> In20_term/1
  Sys_mode/1 -> Compare To Constant2/1, Compare To Constant1/1
  Compare To Constant1/1 -> Req1/1
  Compare To Constant2/1 -> Req1/2
  Req1/1 -> Prop1/1

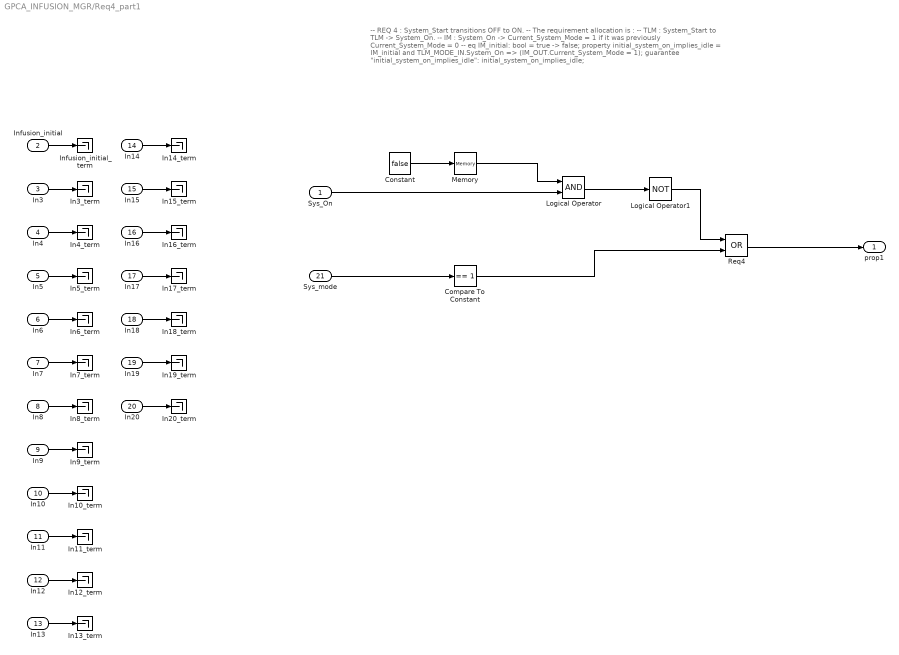
== system GPCA_INFUSION_MGR/Req4_part1 ==
  note: -- REQ 4 : System_Start transitions OFF to ON.
      | -- The requirement allocation is :
      | -- TLM : System_Start to TLM -> System_On.
      | -- IM : System_On -> Current_System_Mode = 1 if it was previously Current_System_Mode = 0
      | --
      | eq IM_initial: bool = true -> false;
      |
      | property initial_system_on_implies_idle =
      | IM_initial and TLM_MODE_IN.System_On => (IM_OUT.Current_System_Mode = 1);
      | guarantee "initial_system_on_implies_idle": initial_system_on_implies_idle;
  Sys_On : Inport
  Infusion_initial : Inport  Port=2
  In3 : Inport  Port=3
  In4 : Inport  Port=4
  In5 : Inport  Port=5
  In6 : Inport  Port=6
  In7 : Inport  Port=7
  In8 : Inport  Port=8
  In9 : Inport  Port=9
  In10 : Inport  Port=10
  In11 : Inport  Port=11
  In12 : Inport  Port=12
  In13 : Inport  Port=13
  In14 : Inport  Port=14
  In15 : Inport  Port=15
  In16 : Inport  Port=16
  In17 : Inport  Port=17
  In18 : Inport  Port=18
  In19 : Inport  Port=19
  In20 : Inport  Port=20
  Sys_mode : Inport  Port=21
  Compare To Constant : simulink/Logic and Bit Operations/Compare To Constant  relop===  const=1  OutDataTypeStr=boolean
  Constant : Constant  Value=false
  In10_term : Terminator
  In11_term : Terminator
  In12_term : Terminator
  In13_term : Terminator
  In14_term : Terminator
  In15_term : Terminator
  In16_term : Terminator
  In17_term : Terminator
  In18_term : Terminator
  In19_term : Terminator
  In20_term : Terminator
  In3_term : Terminator
  In4_term : Terminator
  In5_term : Terminator
  In6_term : Terminator
  In7_term : Terminator
  In8_term : Terminator
  In9_term : Terminator
  Infusion_initial_term : Terminator
  Logical Operator : Logic  AllPortsSameDT=off  OutDataTypeStr=boolean
  Logical Operator1 : Logic  Operator=NOT  AllPortsSameDT=off  OutDataTypeStr=boolean
  Memory : Memory  X0=true
  Req4 : Logic  Operator=OR  AllPortsSameDT=off  OutDataTypeStr=boolean
  prop1 : Outport
  wires:
  Sys_On/1 -> Logical Operator/2
  Infusion_initial/1 -> Infusion_initial_term/1
  In3/1 -> In3_term/1
  In4/1 -> In4_term/1
  In5/1 -> In5_term/1
  In6/1 -> In6_term/1
  In7/1 -> In7_term/1
  In8/1 -> In8_term/1
  In9/1 -> In9_term/1
  In10/1 -> In10_term/1
  In11/1 -> In11_term/1
  In12/1 -> In12_term/1
  In13/1 -> In13_term/1
  In14/1 -> In14_term/1
  In15/1 -> In15_term/1
  In16/1 -> In16_term/1
  In17/1 -> In17_term/1
  In18/1 -> In18_term/1
  In19/1 -> In19_term/1
  In20/1 -> In20_term/1
  Sys_mode/1 -> Compare To Constant/1
  Constant/1 -> Memory/1
  Memory/1 -> Logical Operator/1
  Logical Operator/1 -> Logical Operator1/1
  Logical Operator1/1 -> Req4/1
  Compare To Constant/1 -> Req4/2
  Req4/1 -> prop1/1

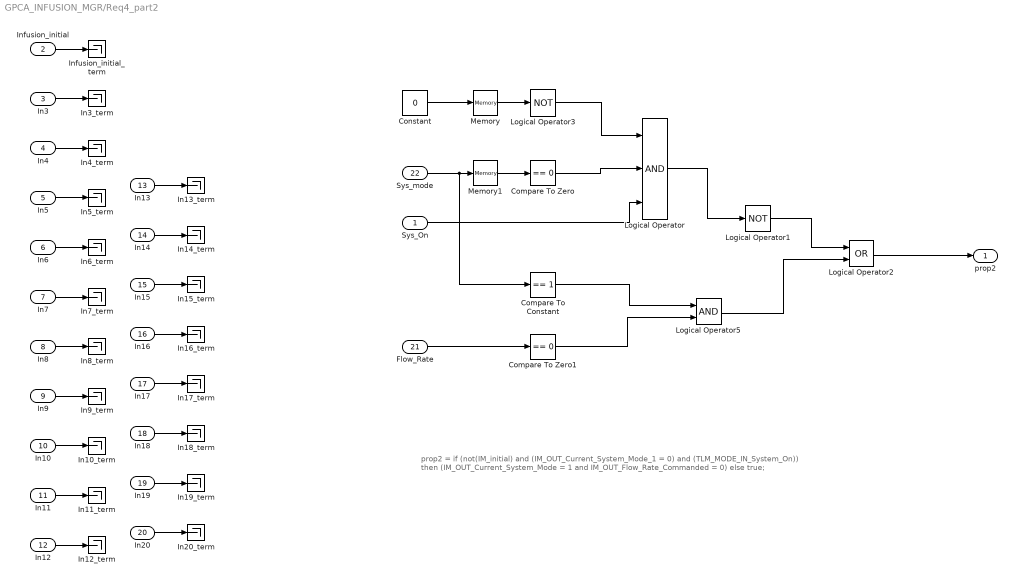
== system GPCA_INFUSION_MGR/Req4_part2 ==
  note: prop2 = if (not(IM_initial) and (IM_OUT_Current_System_Mode_1 = 0) and (TLM_MODE_IN_System_On))
      | then (IM_OUT_Current_System_Mode = 1 and IM_OUT_Flow_Rate_Commanded = 0) else true;
  Sys_On : Inport
  Infusion_initial : Inport  Port=2
  In3 : Inport  Port=3
  In4 : Inport  Port=4
  In5 : Inport  Port=5
  In6 : Inport  Port=6
  In7 : Inport  Port=7
  In8 : Inport  Port=8
  In9 : Inport  Port=9
  In10 : Inport  Port=10
  In11 : Inport  Port=11
  In12 : Inport  Port=12
  In13 : Inport  Port=13
  In14 : Inport  Port=14
  In15 : Inport  Port=15
  In16 : Inport  Port=16
  In17 : Inport  Port=17
  In18 : Inport  Port=18
  In19 : Inport  Port=19
  In20 : Inport  Port=20
  Flow_Rate : Inport  Port=21
  Sys_mode : Inport  Port=22
  Compare To Constant : simulink/Logic and Bit Operations/Compare To Constant  relop===  const=1  OutDataTypeStr=boolean
  Compare To Zero : simulink/Logic and Bit Operations/Compare To Zero  relop===  OutDataTypeStr=boolean
  Compare To Zero1 : simulink/Logic and Bit Operations/Compare To Zero  relop===  OutDataTypeStr=boolean
  Constant : Constant  Value=0
  In10_term : Terminator
  In11_term : Terminator
  In12_term : Terminator
  In13_term : Terminator
  In14_term : Terminator
  In15_term : Terminator
  In16_term : Terminator
  In17_term : Terminator
  In18_term : Terminator
  In19_term : Terminator
  In20_term : Terminator
  In3_term : Terminator
  In4_term : Terminator
  In5_term : Terminator
  In6_term : Terminator
  In7_term : Terminator
  In8_term : Terminator
  In9_term : Terminator
  Infusion_initial_term : Terminator
  Logical Operator : Logic  Inputs=3  AllPortsSameDT=off  OutDataTypeStr=boolean
  Logical Operator1 : Logic  Operator=NOT  AllPortsSameDT=off  OutDataTypeStr=boolean
  Logical Operator2 : Logic  Operator=OR  AllPortsSameDT=off  OutDataTypeStr=boolean
  Logical Operator3 : Logic  Operator=NOT  AllPortsSameDT=off  OutDataTypeStr=boolean
  Logical Operator5 : Logic  AllPortsSameDT=off  OutDataTypeStr=boolean
  Memory : Memory  X0=1
  Memory1 : Memory
  prop2 : Outport
  wires:
  Sys_On/1 -> Logical Operator/3
  Infusion_initial/1 -> Infusion_initial_term/1
  In3/1 -> In3_term/1
  In4/1 -> In4_term/1
  In5/1 -> In5_term/1
  In6/1 -> In6_term/1
  In7/1 -> In7_term/1
  In8/1 -> In8_term/1
  In9/1 -> In9_term/1
  In10/1 -> In10_term/1
  In11/1 -> In11_term/1
  In12/1 -> In12_term/1
  In13/1 -> In13_term/1
  In14/1 -> In14_term/1
  In15/1 -> In15_term/1
  In16/1 -> In16_term/1
  In17/1 -> In17_term/1
  In18/1 -> In18_term/1
  In19/1 -> In19_term/1
  In20/1 -> In20_term/1
  Flow_Rate/1 -> Compare To Zero1/1
  Compare To Zero/1 -> Logical Operator/2
  Sys_mode/1 -> Compare To Constant/1, Memory1/1
  Constant/1 -> Memory/1
  Logical Operator1/1 -> Logical Operator2/1
  Logical Operator2/1 -> prop2/1
  Memory/1 -> Logical Operator3/1
  Logical Operator3/1 -> Logical Operator/1
  Logical Operator/1 -> Logical Operator1/1
  Compare To Constant/1 -> Logical Operator5/1
  Compare To Zero1/1 -> Logical Operator5/2
  Logical Operator5/1 -> Logical Operator2/2
  Memory1/1 -> Compare To Zero/1

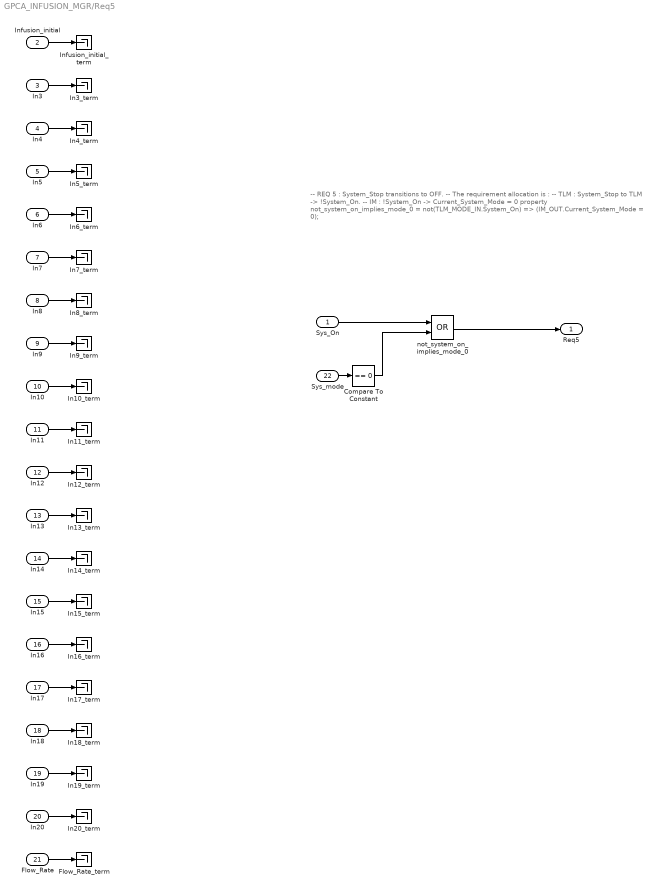
== system GPCA_INFUSION_MGR/Req5 ==
  note: -- REQ 5 : System_Stop transitions to OFF.
      | -- The requirement allocation is :
      | -- TLM : System_Stop to TLM -> !System_On.
      | -- IM : !System_On -> Current_System_Mode = 0
      |
      | property not_system_on_implies_mode_0 =
      | not(TLM_MODE_IN.System_On) => (IM_OUT.Current_System_Mode = 0);
  Sys_On : Inport
  Infusion_initial : Inport  Port=2
  In3 : Inport  Port=3
  In4 : Inport  Port=4
  In5 : Inport  Port=5
  In6 : Inport  Port=6
  In7 : Inport  Port=7
  In8 : Inport  Port=8
  In9 : Inport  Port=9
  In10 : Inport  Port=10
  In11 : Inport  Port=11
  In12 : Inport  Port=12
  In13 : Inport  Port=13
  In14 : Inport  Port=14
  In15 : Inport  Port=15
  In16 : Inport  Port=16
  In17 : Inport  Port=17
  In18 : Inport  Port=18
  In19 : Inport  Port=19
  In20 : Inport  Port=20
  Flow_Rate : Inport  Port=21
  Sys_mode : Inport  Port=22
  Compare To Constant : simulink/Logic and Bit Operations/Compare To Constant  relop===  const=0  OutDataTypeStr=boolean
  Flow_Rate_term : Terminator
  In10_term : Terminator
  In11_term : Terminator
  In12_term : Terminator
  In13_term : Terminator
  In14_term : Terminator
  In15_term : Terminator
  In16_term : Terminator
  In17_term : Terminator
  In18_term : Terminator
  In19_term : Terminator
  In20_term : Terminator
  In3_term : Terminator
  In4_term : Terminator
  In5_term : Terminator
  In6_term : Terminator
  In7_term : Terminator
  In8_term : Terminator
  In9_term : Terminator
  Infusion_initial_term : Terminator
  not_system_on_implies_mode_0 : Logic  Operator=OR  AllPortsSameDT=off  OutDataTypeStr=boolean
  Req5 : Outport
  wires:
  Sys_On/1 -> not_system_on_implies_mode_0/1
  Infusion_initial/1 -> Infusion_initial_term/1
  In3/1 -> In3_term/1
  In4/1 -> In4_term/1
  In5/1 -> In5_term/1
  In6/1 -> In6_term/1
  In7/1 -> In7_term/1
  In8/1 -> In8_term/1
  In9/1 -> In9_term/1
  In10/1 -> In10_term/1
  In11/1 -> In11_term/1
  In12/1 -> In12_term/1
  In13/1 -> In13_term/1
  In14/1 -> In14_term/1
  In15/1 -> In15_term/1
  In16/1 -> In16_term/1
  In17/1 -> In17_term/1
  In18/1 -> In18_term/1
  In19/1 -> In19_term/1
  In20/1 -> In20_term/1
  Flow_Rate/1 -> Flow_Rate_term/1
  Sys_mode/1 -> Compare To Constant/1
  Compare To Constant/1 -> not_system_on_implies_mode_0/2
  not_system_on_implies_mode_0/1 -> Req5/1

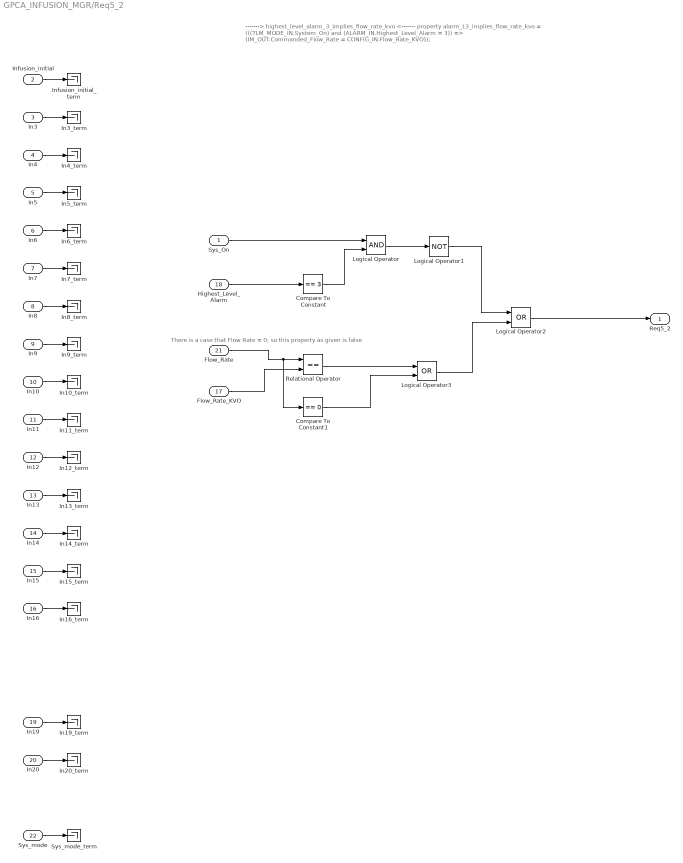
== system GPCA_INFUSION_MGR/Req5_2 ==
  note: There is a case that Flow Rate = 0; so this property as given is false
  note: -------> highest_level_alarm_3_implies_flow_rate_kvo <-------
      |
      | property alarm_L3_implies_flow_rate_kvo =
      | (((TLM_MODE_IN.System_On) and (ALARM_IN.Highest_Level_Alarm = 3)) => (IM_OUT.Commanded_Flow_Rate = CONFIG_IN.Flow_Rate_KVO));
  Sys_On : Inport
  Infusion_initial : Inport  Port=2
  In3 : Inport  Port=3
  In4 : Inport  Port=4
  In5 : Inport  Port=5
  In6 : Inport  Port=6
  In7 : Inport  Port=7
  In8 : Inport  Port=8
  In9 : Inport  Port=9
  In10 : Inport  Port=10
  In11 : Inport  Port=11
  In12 : Inport  Port=12
  In13 : Inport  Port=13
  In14 : Inport  Port=14
  In15 : Inport  Port=15
  In16 : Inport  Port=16
  Flow_Rate_KVO : Inport  Port=17
  Highest_Level_Alarm : Inport  Port=18
  In19 : Inport  Port=19
  In20 : Inport  Port=20
  Flow_Rate : Inport  Port=21
  Sys_mode : Inport  Port=22
  Compare To Constant : simulink/Logic and Bit Operations/Compare To Constant  relop===  const=3  OutDataTypeStr=boolean
  Compare To Constant1 : simulink/Logic and Bit Operations/Compare To Constant  relop===  const=0  OutDataTypeStr=boolean
  In10_term : Terminator
  In11_term : Terminator
  In12_term : Terminator
  In13_term : Terminator
  In14_term : Terminator
  In15_term : Terminator
  In16_term : Terminator
  In19_term : Terminator
  In20_term : Terminator
  In3_term : Terminator
  In4_term : Terminator
  In5_term : Terminator
  In6_term : Terminator
  In7_term : Terminator
  In8_term : Terminator
  In9_term : Terminator
  Infusion_initial_term : Terminator
  Logical Operator : Logic  AllPortsSameDT=off  OutDataTypeStr=boolean
  Logical Operator1 : Logic  Operator=NOT  AllPortsSameDT=off  OutDataTypeStr=boolean
  Logical Operator2 : Logic  Operator=OR  AllPortsSameDT=off  OutDataTypeStr=boolean
  Logical Operator3 : Logic  Operator=OR  AllPortsSameDT=off  OutDataTypeStr=boolean
  Relational Operator : RelationalOperator  Operator===  OutDataTypeStr=boolean
  Sys_mode_term : Terminator
  Req5_2 : Outport
  wires:
  Sys_On/1 -> Logical Operator/1
  Infusion_initial/1 -> Infusion_initial_term/1
  In3/1 -> In3_term/1
  In4/1 -> In4_term/1
  In5/1 -> In5_term/1
  In6/1 -> In6_term/1
  In7/1 -> In7_term/1
  In8/1 -> In8_term/1
  In9/1 -> In9_term/1
  In10/1 -> In10_term/1
  In11/1 -> In11_term/1
  In12/1 -> In12_term/1
  In13/1 -> In13_term/1
  In14/1 -> In14_term/1
  In15/1 -> In15_term/1
  In16/1 -> In16_term/1
  Flow_Rate_KVO/1 -> Relational Operator/2
  Highest_Level_Alarm/1 -> Compare To Constant/1
  In19/1 -> In19_term/1
  In20/1 -> In20_term/1
  Flow_Rate/1 -> Compare To Constant1/1, Relational Operator/1
  Sys_mode/1 -> Sys_mode_term/1
  Compare To Constant/1 -> Logical Operator/2
  Logical Operator/1 -> Logical Operator1/1
  Logical Operator1/1 -> Logical Operator2/1
  Relational Operator/1 -> Logical Operator3/1
  Logical Operator2/1 -> Req5_2/1
  Logical Operator3/1 -> Logical Operator2/2
  Compare To Constant1/1 -> Logical Operator3/2

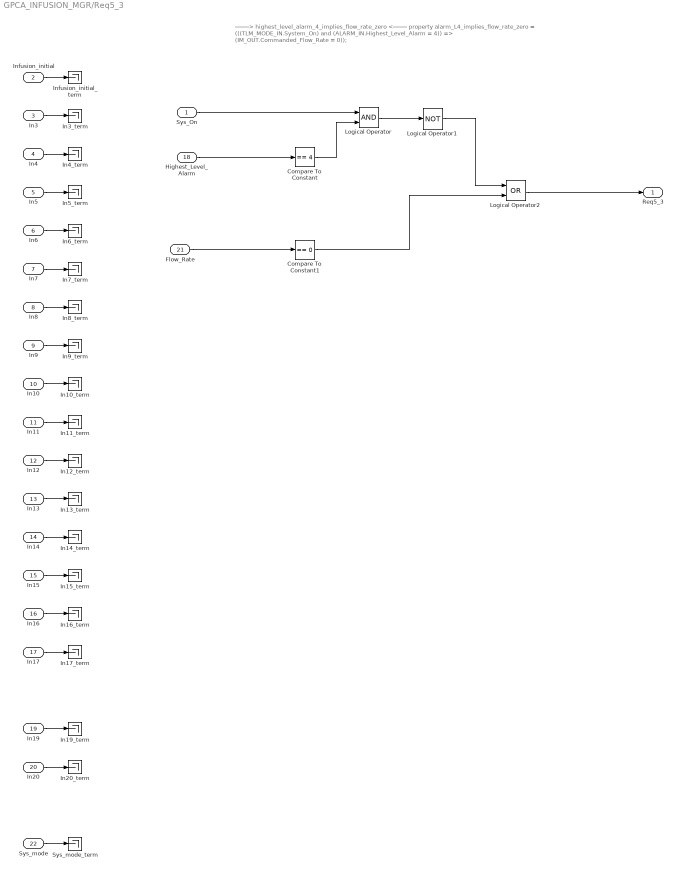
== system GPCA_INFUSION_MGR/Req5_3 ==
  note: -------> highest_level_alarm_4_implies_flow_rate_zero <-------
      |
      | property alarm_L4_implies_flow_rate_zero =
      | (((TLM_MODE_IN.System_On) and (ALARM_IN.Highest_Level_Alarm = 4)) => (IM_OUT.Commanded_Flow_Rate = 0));
  Sys_On : Inport
  Infusion_initial : Inport  Port=2
  In3 : Inport  Port=3
  In4 : Inport  Port=4
  In5 : Inport  Port=5
  In6 : Inport  Port=6
  In7 : Inport  Port=7
  In8 : Inport  Port=8
  In9 : Inport  Port=9
  In10 : Inport  Port=10
  In11 : Inport  Port=11
  In12 : Inport  Port=12
  In13 : Inport  Port=13
  In14 : Inport  Port=14
  In15 : Inport  Port=15
  In16 : Inport  Port=16
  In17 : Inport  Port=17
  Highest_Level_Alarm : Inport  Port=18
  In19 : Inport  Port=19
  In20 : Inport  Port=20
  Flow_Rate : Inport  Port=21
  Sys_mode : Inport  Port=22
  Compare To Constant : simulink/Logic and Bit Operations/Compare To Constant  relop===  const=4  OutDataTypeStr=boolean
  Compare To Constant1 : simulink/Logic and Bit Operations/Compare To Constant  relop===  const=0  OutDataTypeStr=boolean
  In10_term : Terminator
  In11_term : Terminator
  In12_term : Terminator
  In13_term : Terminator
  In14_term : Terminator
  In15_term : Terminator
  In16_term : Terminator
  In17_term : Terminator
  In19_term : Terminator
  In20_term : Terminator
  In3_term : Terminator
  In4_term : Terminator
  In5_term : Terminator
  In6_term : Terminator
  In7_term : Terminator
  In8_term : Terminator
  In9_term : Terminator
  Infusion_initial_term : Terminator
  Logical Operator : Logic  AllPortsSameDT=off  OutDataTypeStr=boolean
  Logical Operator1 : Logic  Operator=NOT  AllPortsSameDT=off  OutDataTypeStr=boolean
  Logical Operator2 : Logic  Operator=OR  AllPortsSameDT=off  OutDataTypeStr=boolean
  Sys_mode_term : Terminator
  Req5_3 : Outport
  wires:
  Infusion_initial/1 -> Infusion_initial_term/1
  In3/1 -> In3_term/1
  In4/1 -> In4_term/1
  In5/1 -> In5_term/1
  In6/1 -> In6_term/1
  In7/1 -> In7_term/1
  In8/1 -> In8_term/1
  In9/1 -> In9_term/1
  In10/1 -> In10_term/1
  In11/1 -> In11_term/1
  In12/1 -> In12_term/1
  In13/1 -> In13_term/1
  In14/1 -> In14_term/1
  In15/1 -> In15_term/1
  In16/1 -> In16_term/1
  In17/1 -> In17_term/1
  In19/1 -> In19_term/1
  In20/1 -> In20_term/1
  Flow_Rate/1 -> Compare To Constant1/1
  Sys_mode/1 -> Sys_mode_term/1
  Sys_On/1 -> Logical Operator/1
  Highest_Level_Alarm/1 -> Compare To Constant/1
  Compare To Constant/1 -> Logical Operator/2
  Logical Operator/1 -> Logical Operator1/1
  Logical Operator1/1 -> Logical Operator2/1
  Logical Operator2/1 -> Req5_3/1
  Compare To Constant1/1 -> Logical Operator2/2

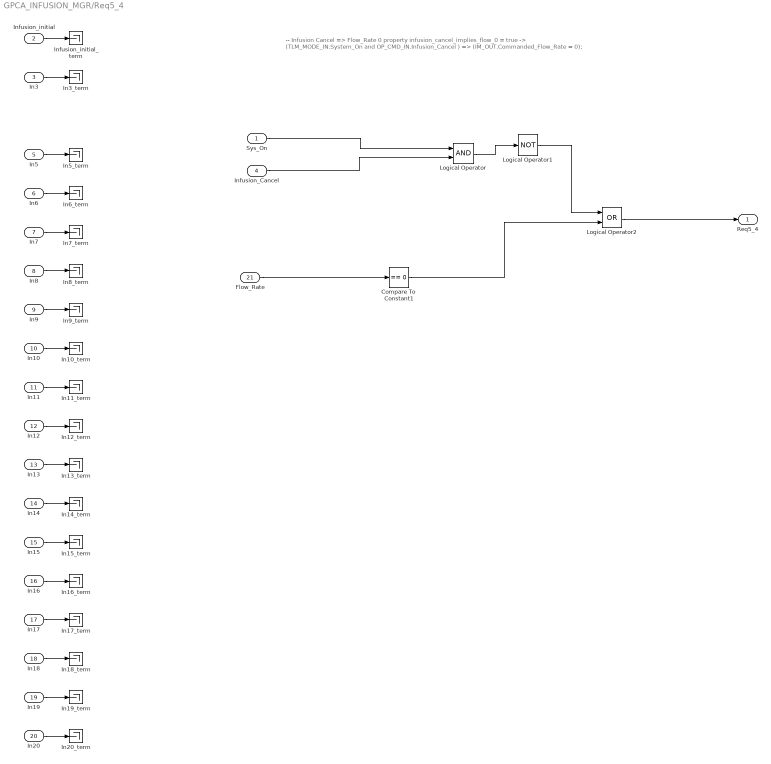
== system GPCA_INFUSION_MGR/Req5_4 ==
  note: -- Infusion Cancel => Flow_Rate 0
      | property infusion_cancel_implies_flow_0 =
      | true ->
      | (TLM_MODE_IN.System_On and OP_CMD_IN.Infusion_Cancel ) =>
      | (IM_OUT.Commanded_Flow_Rate = 0);
  Sys_On : Inport
  Infusion_initial : Inport  Port=2
  In3 : Inport  Port=3
  Infusion_Cancel : Inport  Port=4
  In5 : Inport  Port=5
  In6 : Inport  Port=6
  In7 : Inport  Port=7
  In8 : Inport  Port=8
  In9 : Inport  Port=9
  In10 : Inport  Port=10
  In11 : Inport  Port=11
  In12 : Inport  Port=12
  In13 : Inport  Port=13
  In14 : Inport  Port=14
  In15 : Inport  Port=15
  In16 : Inport  Port=16
  In17 : Inport  Port=17
  In18 : Inport  Port=18
  In19 : Inport  Port=19
  In20 : Inport  Port=20
  Flow_Rate : Inport  Port=21
  Compare To Constant1 : simulink/Logic and Bit Operations/Compare To Constant  relop===  const=0  OutDataTypeStr=boolean
  In10_term : Terminator
  In11_term : Terminator
  In12_term : Terminator
  In13_term : Terminator
  In14_term : Terminator
  In15_term : Terminator
  In16_term : Terminator
  In17_term : Terminator
  In18_term : Terminator
  In19_term : Terminator
  In20_term : Terminator
  In3_term : Terminator
  In5_term : Terminator
  In6_term : Terminator
  In7_term : Terminator
  In8_term : Terminator
  In9_term : Terminator
  Infusion_initial_term : Terminator
  Logical Operator : Logic  AllPortsSameDT=off  OutDataTypeStr=boolean
  Logical Operator1 : Logic  Operator=NOT  AllPortsSameDT=off  OutDataTypeStr=boolean
  Logical Operator2 : Logic  Operator=OR  AllPortsSameDT=off  OutDataTypeStr=boolean
  Req5_4 : Outport
  wires:
  Infusion_initial/1 -> Infusion_initial_term/1
  In3/1 -> In3_term/1
  Infusion_Cancel/1 -> Logical Operator/2
  In5/1 -> In5_term/1
  In6/1 -> In6_term/1
  In7/1 -> In7_term/1
  In8/1 -> In8_term/1
  In9/1 -> In9_term/1
  In10/1 -> In10_term/1
  In11/1 -> In11_term/1
  In12/1 -> In12_term/1
  In13/1 -> In13_term/1
  In14/1 -> In14_term/1
  In15/1 -> In15_term/1
  In16/1 -> In16_term/1
  In17/1 -> In17_term/1
  In18/1 -> In18_term/1
  In19/1 -> In19_term/1
  In20/1 -> In20_term/1
  Flow_Rate/1 -> Compare To Constant1/1
  Sys_On/1 -> Logical Operator/1
  Logical Operator/1 -> Logical Operator1/1
  Logical Operator1/1 -> Logical Operator2/1
  Logical Operator2/1 -> Req5_4/1
  Compare To Constant1/1 -> Logical Operator2/2

== stateflow chart Infusion MGR ==
  state NOT_ON
    entry: IM_OUT_Current_System_Mode=0;
    IM_OUT_Flow_Rate_Commanded=0;
    during: IM_OUT_Current_System_Mode=0;
    IM_OUT_Flow_Rate_Commanded=0;
    exit:IM_OUT_Current_System_Mode=0;
    IM_OUT_Flow_Rate_Commanded=0;
  state Infusion_Manager
    state THERAPY
      during: IM_OUT_New_Infusion=0;
      exit:TherapyExitOperations();
      state ACTIVE
        state Arbiter [parallel]
          settings: executionOrder=4
          state Patient_Bolus
            entry: IM_OUT_Flow_Rate_Commanded=CONFIG_IN_Flow_Rate_Patient_Bolus;
            IM_OUT_Current_System_Mode=4;
            during: IM_OUT_Flow_Rate_Commanded=CONFIG_IN_Flow_Rate_Patient_Bolus;
            IM_OUT_Current_System_Mode=4;
          state Intermittent_Bolus
            entry: IM_OUT_Flow_Rate_Commanded=CONFIG_IN_Flow_Rate_Intermittent_Bolus;
            IM_OUT_Current_System_Mode=3;
            during: IM_OUT_Flow_Rate_Commanded=CONFIG_IN_Flow_Rate_Intermittent_Bolus;
            IM_OUT_Current_System_Mode=3;
          state Basal
            entry:IM_OUT_Flow_Rate_Commanded=CONFIG_IN_Flow_Rate_Basal;
            IM_OUT_Current_System_Mode=2;
            during:IM_OUT_Flow_Rate_Commanded=CONFIG_IN_Flow_Rate_Basal;
            IM_OUT_Current_System_Mode=2;
          (default) -> (junction 54)
          (junction 54) -> Patient_Bolus [order 1] : [in(PATIENT.ON)]
          (junction 54) -> Intermittent_Bolus [order 2] : [in(INTERMITTENT.ON)]
          (junction 54) -> Basal [order 3]
          (junction 55) -> (junction 54)
          Patient_Bolus -> (junction 56)
          Intermittent_Bolus -> (junction 56)
          Basal -> (junction 56)
          (junction 56) -> (junction 55) : {IM_OUT_Actual_Infusion_Duration++}
        state BASAL [parallel]
          settings: executionOrder=1
          state ON
          state OFF
          (default) -> Infusion_Manager.THERAPY.ACTIVE.BASAL.ON
          Infusion_Manager.THERAPY.ACTIVE.BASAL.OFF -> Infusion_Manager.THERAPY.ACTIVE.BASAL.ON : [OP_CMD_IN_Infusion_Initiate]
          Infusion_Manager.THERAPY.ACTIVE.BASAL.ON -> Infusion_Manager.THERAPY.ACTIVE.BASAL.OFF : [IM_OUT_Actual_Infusion_Duration >= Step_Scaling_Factor(CONFIG_IN_Infusion_Total_Duration-1,step_size)]
        state PATIENT [parallel]
          settings: executionOrder=2
          state ON
            entry:number_pbolus++;
            inPatientBolus=1;
            pbolus_timer++;
            IM_OUT_Is_Locked_Out=false;
            during: pbolus_timer++;
            exit: pbolus_timer++;
          state OFF
            entry:pbolus_timer=0;
            inPatientBolus=0;
            IM_OUT_Is_Locked_Out=false;
          state LOCKOUT
            entry:IM_OUT_Lock_Timer++;
            IM_OUT_Is_Locked_Out=true;
            during:IM_OUT_Is_Locked_Out=true;
            IM_OUT_Lock_Timer++;
          (default) -> Infusion_Manager.THERAPY.ACTIVE.PATIENT.OFF [order 2]
          Infusion_Manager.THERAPY.ACTIVE.PATIENT.OFF -> Infusion_Manager.THERAPY.ACTIVE.PATIENT.ON : [PATIENT_IN_Patient_Bolus_Request  && ALARM_IN_Highest_Level_Alarm < 2 && number_pbolus<CONFIG_IN_Max_Number_of_Patient_Bolus ]
          Infusion_Manager.THERAPY.ACTIVE.PATIENT.ON -> LOCKOUT : [pbolus_timer >= Step_Scaling_Factor(CONFIG_IN_Duration_Patient_Bolus-1, step_size) || ALARM_IN_Highest_Level_Alarm == 2]{IM_OUT_Lock_Timer=0;}
          LOCKOUT -> Infusion_Manager.THERAPY.ACTIVE.PATIENT.OFF : [IM_OUT_Lock_Timer >= Step_Scaling_Factor(CONFIG_IN_Lockout_Period_Patient_Bolus-1,step_size)]
          (default) -> LOCKOUT [order 1] : [inPatientBolus]
        state INTERMITTENT [parallel]
          entry: sbolusInter_timer++;
          during : sbolusInter_timer++;
          settings: executionOrder=3
          state ON
            during: sbolus_timer++;
            sbolus_req=0;
            exit: sbolus_timer++;
            sbolus_req=0;
          state OFF
            entry:sbolus_timer=0;
            sbolus_req= sbolus_trigger(sbolusInter_timer, CONFIG_IN_Interval_Intermittent_Bolus, step_size);
            sbolus_trigger2(sbolus_req);
            during: sbolus_req= sbolus_trigger(sbolusInter_timer, CONFIG_IN_Interval_Intermittent_Bolus, step_size);
            sbolus_trigger2(sbolus_req);
            state sbolus_trigger2(sb) [function]
              (default) -> (junction 78) : [sb==1]{sbolusInter_timer=0;}
          (default) -> Infusion_Manager.THERAPY.ACTIVE.INTERMITTENT.OFF
          Infusion_Manager.THERAPY.ACTIVE.INTERMITTENT.OFF -> Infusion_Manager.THERAPY.ACTIVE.INTERMITTENT.ON : [sbolus_req  && ALARM_IN_Highest_Level_Alarm < 2 ]
          Infusion_Manager.THERAPY.ACTIVE.INTERMITTENT.ON -> Infusion_Manager.THERAPY.ACTIVE.INTERMITTENT.OFF : [sbolus_timer >= Step_Scaling_Factor(CONFIG_IN_Duration_Intermittent_Bolus-1,step_size) || ALARM_IN_Highest_Level_Alarm == 2]
        state sb= sbolus_trigger(sbolusInter_timer, CONFIG_IN_Interval_Intermittent_Bolus, step_size) [function]
          (default) -> (junction 84) : {sb = 0;}
          (junction 84) -> (junction 85) [order 1] : [sbolusInter_timer > Step_Scaling_Factor(CONFIG_IN_Interval_Intermittent_Bolus, step_size) || sbolusInter_timer < Step_Scaling_Factor(CONFIG_IN_Interval_Intermittent_Bolus, step_size) ]{sb = 0;}
          (junction 84) -> (junction 86) [order 2] : [sbolusInter_timer == Step_Scaling_Factor(CONFIG_IN_Interval_Intermittent_Bolus, step_size)] {sb = 1;}
      state PAUSED
        state Arbiter [parallel]
          settings: executionOrder=3
          state Paused_NoKVO
            entry: IM_OUT_Flow_Rate_Commanded =0;
            IM_OUT_Current_System_Mode=6;
            during: IM_OUT_Flow_Rate_Commanded =0;
            IM_OUT_Current_System_Mode=6;
            exit: IM_OUT_Flow_Rate_Commanded =0;
            IM_OUT_Current_System_Mode=6;
          state Paused_KVO
            entry: IM_OUT_Flow_Rate_Commanded =CONFIG_IN_Flow_Rate_KVO;
            IM_OUT_Current_System_Mode=7;
            during: IM_OUT_Flow_Rate_Commanded =CONFIG_IN_Flow_Rate_KVO;
            IM_OUT_Current_System_Mode=7;
            exit: IM_OUT_Flow_Rate_Commanded =CONFIG_IN_Flow_Rate_KVO;
            IM_OUT_Current_System_Mode=7;
          state Manual_Paused_KVO
            entry:IM_OUT_Flow_Rate_Commanded=CONFIG_IN_Flow_Rate_KVO;
            IM_OUT_Current_System_Mode=8;
            during:IM_OUT_Flow_Rate_Commanded=CONFIG_IN_Flow_Rate_KVO;
            IM_OUT_Current_System_Mode=8;
            exit:IM_OUT_Flow_Rate_Commanded=CONFIG_IN_Flow_Rate_KVO;
            IM_OUT_Current_System_Mode=8;
          (default) -> (junction 90)
          (junction 90) -> Paused_NoKVO [order 1] : [in(Alarm_Paused.ON) && ALARM_IN_Highest_Level_Alarm == 4]
          (junction 90) -> Paused_KVO [order 2] : [in(Alarm_Paused.ON) && ALARM_IN_Highest_Level_Alarm == 3]
          (junction 90) -> Manual_Paused_KVO [order 3]
          (junction 91) -> (junction 90)
          Paused_NoKVO -> (junction 92)
          Paused_KVO -> (junction 92)
          Manual_Paused_KVO -> (junction 92)
          (junction 92) -> (junction 91)
        state Alarm_Paused [parallel]
          settings: executionOrder=1
          state OFF
          state ON
          (default) -> Infusion_Manager.THERAPY.PAUSED.Alarm_Paused.OFF [order 2]
          (default) -> Infusion_Manager.THERAPY.PAUSED.Alarm_Paused.ON [order 1] : [ALARM_IN_Highest_Level_Alarm >= 3]
          Infusion_Manager.THERAPY.PAUSED.Alarm_Paused.OFF -> Infusion_Manager.THERAPY.PAUSED.Alarm_Paused.ON : [ALARM_IN_Highest_Level_Alarm >= 3]
          Infusion_Manager.THERAPY.PAUSED.Alarm_Paused.ON -> Infusion_Manager.THERAPY.PAUSED.Alarm_Paused.OFF : [OP_CMD_IN_Infusion_Initiate && ALARM_IN_Highest_Level_Alarm < 3]
        state Manual_Paused [parallel]
          settings: executionOrder=2
          state OFF
          state ON
          (default) -> Infusion_Manager.THERAPY.PAUSED.Manual_Paused.OFF [order 2]
          (default) -> Infusion_Manager.THERAPY.PAUSED.Manual_Paused.ON [order 1] : [OP_CMD_IN_Infusion_Inhibit]
          Infusion_Manager.THERAPY.PAUSED.Manual_Paused.OFF -> Infusion_Manager.THERAPY.PAUSED.Manual_Paused.ON : [OP_CMD_IN_Infusion_Inhibit]
          Infusion_Manager.THERAPY.PAUSED.Manual_Paused.ON -> Infusion_Manager.THERAPY.PAUSED.Manual_Paused.OFF : [OP_CMD_IN_Infusion_Initiate && !OP_CMD_IN_Infusion_Inhibit]
      state TherapyExitOperations [function]
        (default) -> (junction 110) : {IM_OUT_Flow_Rate_Commanded=0;
            | IM_OUT_New_Infusion=0;
            | IM_OUT_Is_Locked_Out=false;}
      (default) -> PAUSED [order 1] : [OP_CMD_IN_Infusion_Inhibit || ALARM_IN_Highest_Level_Alarm >= 3]
      (default) -> ACTIVE [order 2]
      ACTIVE -> PAUSED : [OP_CMD_IN_Infusion_Inhibit || ALARM_IN_Highest_Level_Alarm >= 3]
      PAUSED -> ACTIVE : [OP_CMD_IN_Infusion_Initiate && ALARM_IN_Highest_Level_Alarm < 3 && !OP_CMD_IN_Infusion_Inhibit]
    state IDLE
      entry:IM_OUT_Current_System_Mode=1;
      IM_OUT_Flow_Rate_Commanded=0;
      resetAllInfusionDetails();
      during :IM_OUT_Current_System_Mode=1;
      IM_OUT_Flow_Rate_Commanded=0;
      exit:IM_OUT_Current_System_Mode=1;
      IM_OUT_Flow_Rate_Commanded=0;
      resetAllInfusionDetails();
    state resetAllInfusionDetails [function]
      (default) -> (junction 112) : {/*resetForNewInfusion();*/
          | IM_OUT_Lock_Timer=0;
          | inPatientBolus=0;
          | number_pbolus=0;
          | IM_OUT_Is_Locked_Out=false;}
    note: From Therapy - you exit, when
        | 1. Infusion complete
        | 2. Infusion is cancelled : Either Volume or Time is reached
        | 3. No Configuration is avaliable
        | 4. Infsuion is tried to be initiated when there no reservoir volume.
        | -- More conditions may need to be added here.
    state sbolus_dur_timer_fun [function]
      (default) -> (junction 114) : {sbolus_dur_timer=0;
          | sbolus_timer=0;
          | pbolus_timer =0;
          | number_pbolus=0;
          | pbolus_dur_timer=0;
          | sbolusInter_timer=0;
          | paused_KVO_timer=0;
          | IM_OUT_Flow_Rate_Commanded=0;
          | IM_OUT_Actual_Infusion_Duration=0;
          | IM_OUT_Is_Locked_Out=false;
          | writeLog(1);}
    (default) -> IDLE
    THERAPY -> (junction 43) [order 1] : [OP_CMD_IN_Infusion_Initiate && CONFIG_IN_Configured ==1 && !SYS_STAT_IN_Reservoir_Empty ] {/*resetForNewInfusion();*/}
    (junction 43) -> THERAPY : {IM_OUT_New_Infusion=1;}
    IDLE -> (junction 43) [order 2] : [OP_CMD_IN_Infusion_Initiate && CONFIG_IN_Configured > 0 && !SYS_STAT_IN_Reservoir_Empty]{resetAllInfusionDetails();}
    THERAPY -> IDLE [order 2] : [IM_OUT_Actual_Infusion_Duration >=  Step_Scaling_Factor(CONFIG_IN_Infusion_Total_Duration-1.0, step_size)  || SYS_STAT_Volume_Infused >= CONFIG_IN_VTBI_Total || (CONFIG_IN_Configured < 1) || (OP_CMD_IN_Infusion_Cancel)]
    IDLE -> IDLE [order 1] : [OP_CMD_IN_Infusion_Cancel]
  state writeLog(logEvent) [function]
    (default) -> (junction 117) : {IM_OUT_Log_Message_ID=logEvent;}
  state returnVal = Step_Scaling_Factor(inputVal, step_size) [function]
    note: This is the operational mode.
    (default) -> (junction 122) : {returnVal=inputVal/step_size;}
  note: step scaling factor returns the scaled time depending upon the step size.
      | If counter has to timeout after 100 seconds and if the step size is 0.1 second
      | the new timeout value = 100/0.1 = 1000 steps.
      | default will be one step = 1 second.
  (default) -> Infusion_Manager [order 1] : [TLM_MODE_IN_System_On]
  (default) -> NOT_ON [order 2]
  NOT_ON -> Infusion_Manager : [TLM_MODE_IN_System_On]
  Infusion_Manager -> NOT_ON : [!TLM_MODE_IN_System_On]
  data: sb function_input boolean; sb function_output boolean; sbolusInter_timer function_input double; CONFIG_IN_Interval_Intermittent_Bolus function_input double; step_size function_input double; logEvent function_input uint8; inputVal function_input double; returnVal function_output double; step_size function_input double; TLM_MODE_IN_System_On input boolean; IM_OUT_Flow_Rate_Commanded output uint8; OP_CMD_IN_Infusion_Initiate input boolean; OP_CMD_IN_Infusion_Inhibit input boolean; OP_CMD_IN_Infusion_Cancel input boolean; sbolus_req local boolean; sbolus_timer local double; pbolus_timer local double; PATIENT_IN_Patient_Bolus_Request input boolean; IM_OUT_Current_System_Mode output uint8; paused_KVO_timer local uint8; CONFIG_IN_Flow_Rate_Basal input uint8; CONFIG_IN_Flow_Rate_Intermittent_Bolus input uint8; CONFIG_IN_Duration_Intermittent_Bolus input double; CONFIG_IN_Flow_Rate_Patient_Bolus input uint8; CONFIG_IN_Duration_Patient_Bolus input double; CONFIG_IN_Lockout_Period_Patient_Bolus input double; sbolus_dur_timer local uint8; pbolus_dur_timer local uint8; IM_OUT_Lock_Timer output double; number_pbolus local uint8; CONFIG_IN_Max_Number_of_Patient_Bolus input uint8; CONFIG_IN_Interval_Intermittent_Bolus input double; CONFIG_IN_Infusion_Total_Duration input double; CONFIG_IN_VTBI_Total input uint8; CONFIG_IN_Configured input uint8; CONFIG_IN_Flow_Rate_KVO input uint8; inPatientBolus local boolean; ALARM_IN_Highest_Level_Alarm input uint8; sbolusInter_timer local double; IM_OUT_New_Infusion output boolean; IM_OUT_Log_Message_ID output uint8; SYS_STAT_IN_Reservoir_Empty input boolean; SYS_STAT_Volume_Infused input uint8; IM_OUT_Actual_Infusion_Duration output double; step_size parameter double; IM_OUT_Is_Locked_Out output boolean
